simulink model "sun"  (R2023a)
settings: Solver=ode4  StartTime=0.0  StopTime=10.0  FixedStep=dt_sun  RelTol=1e-3
settings Model: Creator=ndelurgio  LastModifiedBy=ndelurgio

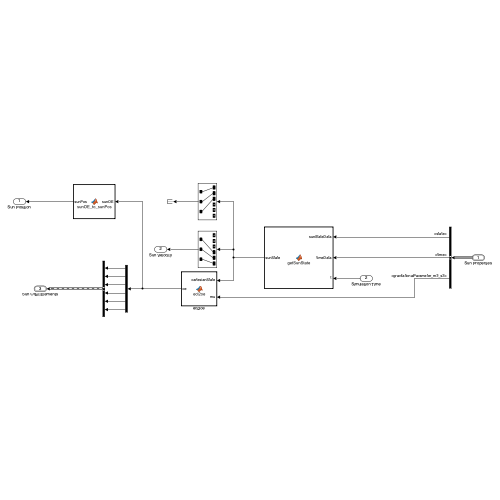
[thumbnail: Simulink's stored preview of the top-level diagram]
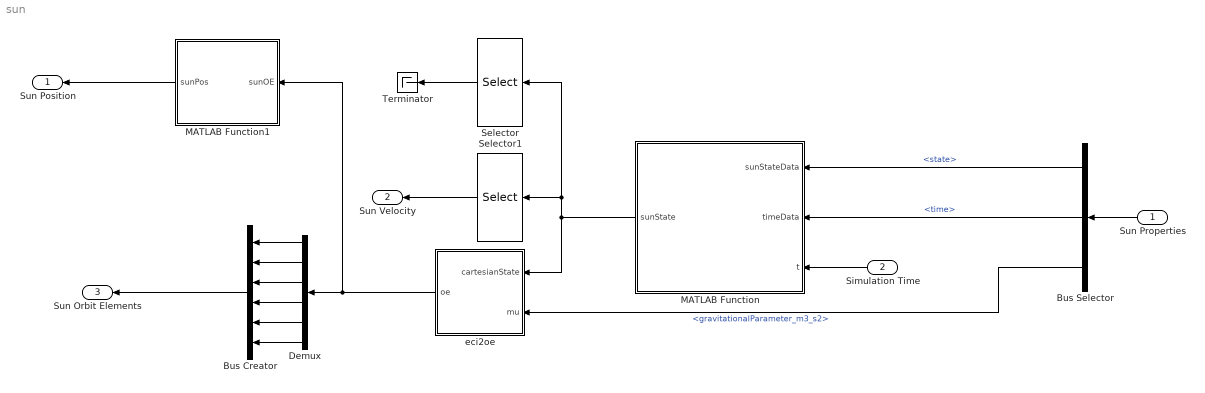
== system sun ==
  Sun Properties : Inport  OutDataTypeStr=Bus: sunProperties
  Simulation Time : Inport  Port=2
  Bus Creator : BusCreator  Inputs=6  OutDataTypeStr=Bus: osculatingOrbitElements  NonVirtualBus=on
      settings: InheritFromInputs=off
  Bus Selector : BusSelector  OutputSignals=state,time,gravitationalParameter_m3_s2
  Demux : Demux  Outputs=6
  MATLAB Function : MATLAB Function  TreatAsAtomicUnit=on
  MATLAB Function1 : MATLAB Function  TreatAsAtomicUnit=on
  Selector : Selector  InputPortWidth=6  IndexOptions=Index vector (dialog)  Indices=[1:3]  OutputSizes=1
  Selector1 : Selector  InputPortWidth=6  IndexOptions=Index vector (dialog)  Indices=[4:6]  OutputSizes=1
  Terminator : Terminator
  eci2oe : MATLAB Function  TreatAsAtomicUnit=on
  Sun Position : Outport
  Sun Velocity : Outport  Port=2
  Sun Orbit Elements : Outport  Port=3  OutDataTypeStr=Bus: osculatingOrbitElements
  wires:
  Sun Properties/1 -> Bus Selector/1
  Bus Selector/1 -> MATLAB Function/1(sunStateData)  "<state>"
  Bus Selector/2 -> MATLAB Function/2(timeData)  "<time>"
  Simulation Time/1 -> MATLAB Function/3(t)
  Selector1/1 -> Sun Velocity/1
  eci2oe/1(oe) -> MATLAB Function1/1(sunOE), Demux/1
  Demux/6 -> Bus Creator/6
  Demux/5 -> Bus Creator/5
  Demux/4 -> Bus Creator/4
  Demux/2 -> Bus Creator/2
  Demux/1 -> Bus Creator/1
  Demux/3 -> Bus Creator/3
  Bus Creator/1 -> Sun Orbit Elements/1
  MATLAB Function/1(sunState) -> Selector1/1, Selector/1, eci2oe/1(cartesianState)
  Bus Selector/3 -> eci2oe/2(mu)  "<gravitationalParameter_m3_s2>"
  Selector/1 -> Terminator/1
  MATLAB Function1/1(sunPos) -> Sun Position/1

== matlab function sun/MATLAB Function ==
  data: sunStateData input; sunState output; timeData input; t input
function sunState = getSunState(sunStateData,timeData,t)

sunState = getSunState(sunStateData,timeData,t);

end

== matlab function sun/eci2oe ==
  data: cartesianState input; oe output; mu input
function oe = eci2oe(cartesianState,mu)
[oe,~,~,~] = eci2oe( cartesianState , mu );
end

== matlab function sun/MATLAB Function1 ==
  data: sunOE input; sunPos output
function sunPos = sunOE_to_sunPos(sunOE)
sunPos = sunOE_to_sunPos(sunOE);
end
